simulink model "ShiojiSimUsingSfunction"  (Simulink 3.00)
settings: Solver=ode45  StartTime=0.0  StopTime=400.0  RelTol=1e-3
libraries: simulink3 x1

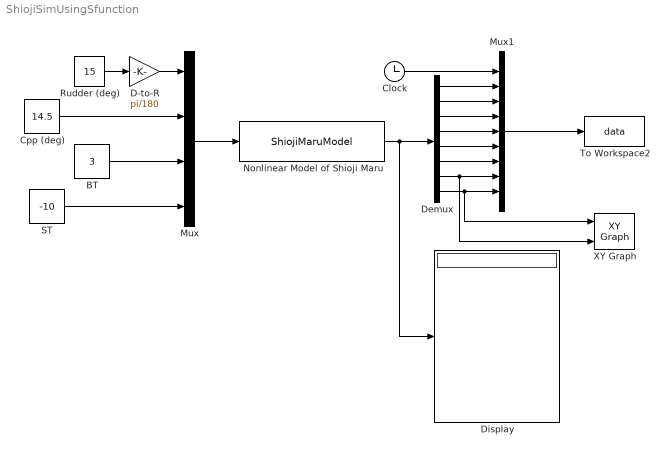
== system ShiojiSimUsingSfunction ==
  BT : Constant  Value=3
  Clock : Clock
      settings: DisplayTime=off  Decimation=10
  Cpp (deg) : Constant  Value=14.5
  D-to-R : Gain  Gain=pi/180  SaturateOnIntegerOverflow=on
  Demux : Demux  Outputs=8
  Display : Display
      settings: Format=short
  Mux : Mux  Inputs=4
  Mux1 : Mux  Inputs=9
  Nonlinear Model of Shioji Maru : S-Function  FunctionName=ShiojiMaruModel  PortCounts=[]  SFunctionModules=''
  Rudder (deg) : Constant  Value=15
  ST : Constant  Value=-10
  To Workspace2 : ToWorkspace  VariableName=data  SampleTime=-1  SaveFormat=Matrix
  XY Graph : simulink3/Sinks/XY Graph  xmin=-100  xmax=500  ymin=-200  ymax=300  st=-1
  wires:
  Nonlinear Model of Shioji Maru/1 -> Display/1, Demux/1
  Mux/1 -> Nonlinear Model of Shioji Maru/1
  Cpp (deg)/1 -> Mux/2
  Rudder (deg)/1 -> D-to-R/1
  D-to-R/1 -> Mux/1
  BT/1 -> Mux/3
  ST/1 -> Mux/4
  Clock/1 -> Mux1/1
  Mux1/1 -> To Workspace2/1
  Demux/7 -> Mux1/8, XY Graph/2
  Demux/8 -> Mux1/9, XY Graph/1
  Demux/6 -> Mux1/7
  Demux/5 -> Mux1/6
  Demux/4 -> Mux1/5
  Demux/3 -> Mux1/4
  Demux/2 -> Mux1/3
  Demux/1 -> Mux1/2
